simulink model "Xcvr_SSB_AM_2p5"  (Simulink 8.0)
settings: Solver=VariableStepDiscrete  SolverMode=SingleTasking  StartTime=0.0  StopTime=10  RelTol=1e-3
PreLoadFcn:
  | Fs=80e6;
  | 
  | phee=da_rom();
  | [phee_1,phee_2]=da_i2_rom();
  | 
  | Dcic=64;       % CIC decimation
  | Dfac=128;    % following DA filter decimation
  | N = 6;           %       (2^(N+1))=Dfac
  | Daudio=Dcic*Dfac;
  | Faudio=Fs/Daudio;
  | 
  | load info_filt_ssb_4
  | load Serial_Intfc_Stream_5
  | 
  | % AGC related
  | x=0.5:1/256:(1-1/256);
  | addr=(x-0.5)*256;
  | y=1./x;
values from neighbouring files (symbols this model uses):
  Serial_Interface = [0 0 0 0 0 0 0 0 0 0 0 0 ... (11390 elements, 2x5695)]    [Serial_Intfc_Stream_5.mat]
undefined symbols (not defined in the file or in its folder): get, sided, Two, xlipgetpartsetting
undefined symbols (not defined in the file): ssb_coef
libraries: xbsIndex_r4 x1305, dspsrcs4 x5, simulink x2, dspsigops x2, dspsnks4 x1
(part 11 of 11)

== system Xcvr_SSB_AM_2p5/Audio_and_Mode_Control/AGC_and_More/AGC Xilinx/Sequential Divide/Shift and lookup ==
  note: Delays to equalize for ROM latency.
  note: b16
  In1 : Inport
  1st 1 detect : Subsystem
  AddSub : xbsIndex_r4/AddSub  mode=Subtraction  use_carryin=off  use_carryout=off  en=off  latency=0  precision=User Defined  arith_type=Unsigned  n_bits=8  bin_pt=0  quantization=Truncate  overflow=Saturate  dbl_ovrd=off  use_behavioral_HDL=off  hw_selection=Fabric  pipelined=off  use_rpm=on  block_type=addsub
      settings: block_version=9.2.00
  AddSub1 : xbsIndex_r4/AddSub  mode=Addition  use_carryin=off  use_carryout=off  en=off  latency=0  precision=User Defined  arith_type=Unsigned  n_bits=8  bin_pt=0  quantization=Truncate  overflow=Saturate  dbl_ovrd=off  use_behavioral_HDL=off  hw_selection=Fabric  pipelined=off  use_rpm=on  block_type=addsub
      settings: block_version=9.2.00
  CMult : xbsIndex_r4/CMult  const=1/8  gui_display_data_type=Fixed-point  const_n_bits=3  const_bin_pt=3  float_type=Single  exp_bits=8  fraction_bits=24  en=off  latency=0  precision=User Defined  arith_type=Unsigned  n_bits=8  bin_pt=0  quantization=Truncate  overflow=Wrap  dbl_ovrd=off  use_behavioral_HDL=off  mem_type=Distributed RAM  pipeline=off  block_type=cmult
      settings: block_version=12.2
  CMult1 : xbsIndex_r4/CMult  const=16  gui_display_data_type=Fixed-point  const_n_bits=5  const_bin_pt=0  float_type=Single  exp_bits=8  fraction_bits=24  en=off  latency=0  precision=User Defined  arith_type=Unsigned  n_bits=8  bin_pt=0  quantization=Truncate  overflow=Wrap  dbl_ovrd=off  use_behavioral_HDL=off  mem_type=Distributed RAM  pipeline=off  block_type=cmult
      settings: block_version=12.2
  Capture Fraction and compute address : Subsystem
  Capture Shift : Subsystem
  Constant : xbsIndex_r4/Constant  const=0  gui_display_data_type=Fixed-point  arith_type=Unsigned  n_bits=5  bin_pt=0  preci_type=Single  exp_width=8  frac_width=24  explicit_period=off  period=1  equ=P=C  opselect=C  inp2=PCIN>>17  opr=+  inp1=P  carry=CIN  dbl_ovrd=off  block_type=constant
      settings: block_version=9.2.00
  Constant1 : xbsIndex_r4/Constant  const=16  gui_display_data_type=Fixed-point  arith_type=Unsigned  n_bits=5  bin_pt=0  preci_type=Single  exp_width=8  frac_width=24  explicit_period=off  period=1  equ=P=C  opselect=C  inp2=PCIN>>17  opr=+  inp1=P  carry=CIN  dbl_ovrd=off  block_type=constant
      settings: block_version=9.2.00
  Constant2 : xbsIndex_r4/Constant  const=15  gui_display_data_type=Fixed-point  arith_type=Unsigned  n_bits=4  bin_pt=0  preci_type=Single  exp_width=8  frac_width=24  explicit_period=off  period=1  equ=P=C  opselect=C  inp2=PCIN>>17  opr=+  inp1=P  carry=CIN  dbl_ovrd=off  block_type=constant
      settings: block_version=9.2.00
  Counter : xbsIndex_r4/Counter  cnt_type=Count Limited  cnt_to=31  operation=Up  start_count=0  cnt_by_val=1  arith_type=Unsigned  n_bits=5  bin_pt=0  load_pin=off  rst=off  en=off  explicit_period=on  period=1/(32*Faudio)  dbl_ovrd=off  use_behavioral_HDL=off  implementation=Fabric  use_rpm=off  block_type=counter
      settings: block_version=9.2.00
  Counter1 : xbsIndex_r4/Counter  cnt_type=Free Running  cnt_to=255  operation=Up  start_count=0  cnt_by_val=1  arith_type=Unsigned  n_bits=8  bin_pt=0  load_pin=off  rst=off  en=off  explicit_period=on  period=1/(32*Faudio)  dbl_ovrd=off  use_behavioral_HDL=off  implementation=Fabric  use_rpm=off  block_type=counter
      settings: block_version=9.2.00
  Delay1 : xbsIndex_r4/Delay  rst=off  infoeditControl=Selection of Reset will increase slice count due to use of real FFs and instead of SRLs  en=off  latency=1  dbl_ovrd=off  reg_retiming=off  block_type=delay
      settings: block_version=9.2.00
  Delay2 : xbsIndex_r4/Delay  rst=off  infoeditControl=Selection of Reset will increase slice count due to use of real FFs and instead of SRLs  en=off  latency=1  dbl_ovrd=off  reg_retiming=off  block_type=delay
      settings: block_version=9.2.00
  Mux : xbsIndex_r4/Mux  inputs=2  en=off  latency=1  precision=Full  arith_type=Unsigned  n_bits=16  bin_pt=14  quantization=Truncate  overflow=Wrap  dbl_ovrd=off  block_type=mux
      settings: block_version=9.2.00
  ROM : xbsIndex_r4/ROM  depth=128  initVector=y  distributed_mem=Block RAM  rst=off  init_reg=0  en=off  latency=1  gui_display_data_type=Fixed-point  arith_type=Unsigned  n_bits=10  bin_pt=9  preci_type=Single  exp_width=8  frac_width=24  dbl_ovrd=off  optimize=Area  use_rpm=on  block_type=sprom
      settings: block_version=9.2.00
  Relational : xbsIndex_r4/Relational  mode=a=b  en=off  latency=0  dbl_ovrd=off  block_type=relational
      settings: block_version=9.2.00
  Relational1 : xbsIndex_r4/Relational  mode=a=b  en=off  latency=0  dbl_ovrd=off  block_type=relational
      settings: block_version=9.2.00
  Relational3 : xbsIndex_r4/Relational  mode=a<b  en=off  latency=0  dbl_ovrd=off  block_type=relational
      settings: block_version=9.2.00
  Shift1 : xbsIndex_r4/Shift  shift_dir=Left  shift_bits=1  en=off  latency=0  precision=User Defined  arith_type=Unsigned  n_bits=16  bin_pt=16  quantization=Truncate  overflow=Wrap  dbl_ovrd=off  block_type=shift
      settings: block_version=9.2.00
  Slice : xbsIndex_r4/Slice  nbits=1  boolean_output=off  mode=Upper Bit Location + Width  bit1=0  base1=MSB of Input  bit0=0  base0=LSB of Input  dbl_ovrd=off  block_type=slice
      settings: infoedit="Extracts a given range of bits from each input sample and presents it at the output.  The output type is ordinarily unsigned with binary point at zero, but can be Boolean when the slice is one bit wide.<P><P>Hardware notes: In hardware this block costs nothing."  block_version=9.2.00
  Ready : Outport
  1/X : Outport  Port=2
  Shift : Outport  Port=3
  Smeter : Outport  Port=4
  wires:
  Delay1/1 -> Ready/1
  ROM/1 -> 1/X/1
  Capture Shift/1(Dout) -> Delay2/1
  Capture Fraction and compute address/1(Dout) -> CMult/1, ROM/1
  1st 1 detect/1(Out1) -> Capture Shift/1(En), Capture Fraction and compute address/2(En)
  Slice/1 -> 1st 1 detect/1(MSbit)
  Relational1/1 -> Delay1/1
  Constant1/1 -> Relational1/2
  Constant/1 -> Relational/2
  Counter/1 -> Capture Shift/2(Din), Relational1/1, Relational/1
  In1/1 -> Mux/3
  Shift1/1 -> Mux/2
  Relational/1 -> 1st 1 detect/2(Rst), Mux/1
  Mux/1 -> Shift1/1, Slice/1, Capture Fraction and compute address/1(Din)
  CMult/1 -> AddSub/2
  AddSub/1 -> Relational3/1
  AddSub1/1 -> AddSub/1
  CMult1/1 -> AddSub1/2
  Constant2/1 -> AddSub1/1
  Delay2/1 -> CMult1/1, Shift/1
  Counter1/1 -> Relational3/2
  Relational3/1 -> Smeter/1  "Uncorrected"

== system Xcvr_SSB_AM_2p5/Audio_and_Mode_Control/AGC_and_More/AGC Xilinx/Sequential Divide/Variable Shifter ==
  EN : Inport
  Din : Inport  Port=2
  Shift in : Inport  Port=3
  Mux : xbsIndex_r4/Mux  inputs=16  en=on  latency=1  precision=Full  arith_type=Unsigned  n_bits=16  bin_pt=14  quantization=Truncate  overflow=Wrap  dbl_ovrd=off  block_type=mux
      settings: block_version=9.2.00
  Shift{1..15} (15 alike) : xbsIndex_r4/Shift  shift_dir=Left  shift_bits=1  en=off  latency=0  precision=Full  arith_type="Signed  (2's comp)"  n_bits=16  bin_pt=14  quantization=Truncate  overflow=Wrap  dbl_ovrd=off  block_type=shift
      settings: block_version=9.2.00
  Out1 : Outport
  wires:
  Shift15/1 -> Mux/17
  Shift14/1 -> Shift15/1, Mux/16
  Shift13/1 -> Shift14/1, Mux/15
  Shift12/1 -> Shift13/1, Mux/14
  Shift11/1 -> Shift12/1, Mux/13
  Shift10/1 -> Shift11/1, Mux/12
  Shift9/1 -> Shift10/1, Mux/11
  Shift8/1 -> Shift9/1, Mux/10
  Shift7/1 -> Shift8/1, Mux/9
  Shift6/1 -> Shift7/1, Mux/8
  Shift5/1 -> Shift6/1, Mux/7
  Shift4/1 -> Shift5/1, Mux/6
  Shift3/1 -> Shift4/1, Mux/5
  Shift2/1 -> Shift3/1, Mux/4
  Shift1/1 -> Shift2/1, Mux/3
  EN/1 -> Mux/18
  Mux/1 -> Out1/1
  Din/1 -> Shift1/1, Mux/2
  Shift in/1 -> Mux/1

== system Xcvr_SSB_AM_2p5/Audio_and_Mode_Control/AGC_and_More/RX_Audio_Filter/n-tap MAC FIR Filter/MAC Engine ==
  note: The precision required for the multiplier and the accumulator is a
      | function of the filter taps (coefficients) and the number of taps. Since
      | these are fixed at design time, it is possible to tailor the hardware resources
      | to the filter specification.  The multiplier need only have enough  bits to
      | compute the product of the largest magnitude coefficient and the largest
      | magnitude data input value.   That is,
      |
      |         mult_nbits = ceil(log2(max(abs(coef*2^coef_binpt))))+input_nbits + 1;
      |         mult_binpt = input_binpt+coef_binpt;
      |
      | Similarly, the accumulator need only have sufficient precision to accumulate
      | maximal input against the filter taps.
      |
      |         acc_nbits = ceil(log2(sum(abs(coef*2^coef_binpt)))) + input_nbits + 1;
      |         acc_binpt = mult_binpt;
      |
      | These variables are passed to the blocks as mask parameters.
  note: Upon reset, the accumulator reinitializes to its current input value
      | rather than zero, which allows the MAC engine to stream data without
      | stalling for one sample period.
  note: This subsystem implements a multiply-accumulate engine.
  note: The Multiplier block is implemented using Virtex-II  dedicated multipliers.
      | Enabling the 'Pipeline to Greatest Extent Possible' mask configuration
      | parameter ensures the internal pipeline stages of the dedicated
      | multipliers are used.
  a : Inport
  b : Inport  Port=2
  rst : Inport  Port=3
  Accumulator : xbsIndex_r4/Accumulator  operation=Add  n_bits=ceil(log2(max(1,sum(abs(coef*2^coef_bin_pt)))))+smpl_n_bits + 1  overflow=Wrap  scale=1  rst=on  infoeditControl=reset for floating point data type must be asserted for a minimum of 2 cycles  hasbypass=on  en=off  latency=0  dbl_ovrd=off  msb_inp=100  msb=100  lsb=-100  use_behavioral_HDL=on  implementation=Fabric  block_type=accum
      settings: infoedit="Adder or subtractor-based accumulator.   Output type and binary point position match the input.<P><P>Hardware notes: When \"Reinitialize with Input 'b' on Reset\" is selected, the accumulator is forced to run at the system rate even if the input 'b' is running at a slower rate."  xl_area=[0, 0, 0, 0, 0, 0, 0]  block_version=VER_STRING_GOES_HERE
  Mult : xbsIndex_r4/Mult  precision=User Defined  arith_type="Signed  (2's comp)"  n_bits=max(ceil(log2(max(1,max(abs(coef*2^coef_bin_pt)))))+smpl_n_bits + 1,smpl_bin_pt+coef_bin_pt)  bin_pt=smpl_bin_pt+coef_bin_pt  quantization=Truncate  overflow=Wrap  en=off  latency=2  dbl_ovrd=off  use_behavioral_HDL=off  opt=Speed  use_embedded=on  optimum_pipeline=off  pipeline=on  use_rpm=on  placement_style=Rectangular shape  block_type=mult
      settings: infoedit=Multiplies two values.<P><P>Hardware notes: To use the internal pipeline stage of the dedicated multiplier you must select 'Pipeline to Greatest Extent Possible'.  xl_area=[0, 0, 0, 0, 0, 0, 0]  block_version=VER_STRING_GOES_HERE
  q : Outport
  wires:
  Mult/1 -> Accumulator/1
  a/1 -> Mult/1
  Accumulator/1 -> q/1
  b/1 -> Mult/2
  rst/1 -> Accumulator/2

== system Xcvr_SSB_AM_2p5/Audio_and_Mode_Control/Audio_Processor/TX Equalizer/n-tap MAC FIR Filter/MAC Engine ==
  note: The precision required for the multiplier and the accumulator is a
      | function of the filter taps (coefficients) and the number of taps. Since
      | these are fixed at design time, it is possible to tailor the hardware resources
      | to the filter specification.  The multiplier need only have enough  bits to
      | compute the product of the largest magnitude coefficient and the largest
      | magnitude data input value.   That is,
      |
      |         mult_nbits = ceil(log2(max(abs(coef*2^coef_binpt))))+input_nbits + 1;
      |         mult_binpt = input_binpt+coef_binpt;
      |
      | Similarly, the accumulator need only have sufficient precision to accumulate
      | maximal input against the filter taps.
      |
      |         acc_nbits = ceil(log2(sum(abs(coef*2^coef_binpt)))) + input_nbits + 1;
      |         acc_binpt = mult_binpt;
      |
      | These variables are passed to the blocks as mask parameters.
  note: Upon reset, the accumulator reinitializes to its current input value
      | rather than zero, which allows the MAC engine to stream data without
      | stalling for one sample period.
  note: This subsystem implements a multiply-accumulate engine.
  note: The Multiplier block is implemented using Virtex-II  dedicated multipliers.
      | Enabling the 'Pipeline to Greatest Extent Possible' mask configuration
      | parameter ensures the internal pipeline stages of the dedicated
      | multipliers are used.
  a : Inport
  b : Inport  Port=2
  rst : Inport  Port=3
  Accumulator : xbsIndex_r4/Accumulator  operation=Add  n_bits=ceil(log2(max(1,sum(abs(coef*2^coef_bin_pt)))))+smpl_n_bits + 1  overflow=Wrap  scale=1  rst=on  infoeditControl=reset for floating point data type must be asserted for a minimum of 2 cycles  hasbypass=on  en=off  latency=0  dbl_ovrd=off  msb_inp=100  msb=100  lsb=-100  use_behavioral_HDL=on  implementation=Fabric  block_type=accum
      settings: infoedit="Adder or subtractor-based accumulator.   Output type and binary point position match the input.<P><P>Hardware notes: When \"Reinitialize with Input 'b' on Reset\" is selected, the accumulator is forced to run at the system rate even if the input 'b' is running at a slower rate."  xl_area=[0, 0, 0, 0, 0, 0, 0]  block_version=VER_STRING_GOES_HERE
  Mult : xbsIndex_r4/Mult  precision=User Defined  arith_type="Signed  (2's comp)"  n_bits=max(ceil(log2(max(1,max(abs(coef*2^coef_bin_pt)))))+smpl_n_bits + 1,smpl_bin_pt+coef_bin_pt)  bin_pt=smpl_bin_pt+coef_bin_pt  quantization=Truncate  overflow=Wrap  en=off  latency=2  dbl_ovrd=off  use_behavioral_HDL=off  opt=Speed  use_embedded=on  optimum_pipeline=off  pipeline=on  use_rpm=on  placement_style=Rectangular shape  block_type=mult
      settings: infoedit=Multiplies two values.<P><P>Hardware notes: To use the internal pipeline stage of the dedicated multiplier you must select 'Pipeline to Greatest Extent Possible'.  xl_area=[0, 0, 0, 0, 0, 0, 0]  block_version=VER_STRING_GOES_HERE
  q : Outport
  wires:
  Mult/1 -> Accumulator/1
  a/1 -> Mult/1
  Accumulator/1 -> q/1
  b/1 -> Mult/2
  rst/1 -> Accumulator/2

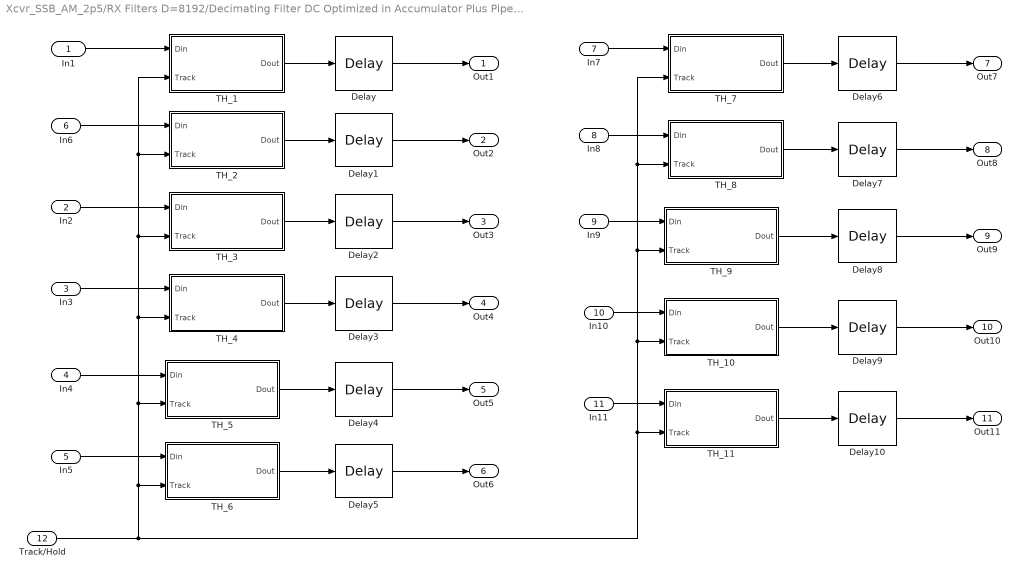
== system Xcvr_SSB_AM_2p5/RX Filters D=8192/Decimating Filter DC Optimized in Accumulator Plus Pipelined Stage Control. Improved dynamic  range. /D=2 Bit Serial Filter Core with Piplined RAM Based SR/RAM Based SR/Track/Hang  Plus 1 Pipe Stage ==
  In1 : Inport
  In2 : Inport  Port=2
  In3 : Inport  Port=3
  In4 : Inport  Port=4
  In5 : Inport  Port=5
  In6 : Inport  Port=6
  In7 : Inport  Port=7
  In8 : Inport  Port=8
  In9 : Inport  Port=9
  In10 : Inport  Port=10
  In11 : Inport  Port=11
  Track/Hold : Inport  Port=12
  Delay{,1..10} (11 alike) : xbsIndex_r4/Delay  rst=off  infoeditControl=Selection of Reset will increase slice count due to use of real FFs and instead of SRLs  en=off  latency=1  dbl_ovrd=off  reg_retiming=off  block_type=delay
      settings: block_version=12.2
  TH_1 : Subsystem
  TH_10 : Subsystem
  TH_11 : Subsystem
  TH_2 : Subsystem
  TH_3 : Subsystem
  TH_4 : Subsystem
  TH_5 : Subsystem
  TH_6 : Subsystem
  TH_7 : Subsystem
  TH_8 : Subsystem
  TH_9 : Subsystem
  Out1 : Outport
  Out2 : Outport  Port=2
  Out3 : Outport  Port=3
  Out4 : Outport  Port=4
  Out5 : Outport  Port=5
  Out6 : Outport  Port=6
  Out7 : Outport  Port=7
  Out8 : Outport  Port=8
  Out9 : Outport  Port=9
  Out10 : Outport  Port=10
  Out11 : Outport  Port=11
  wires:
  TH_5/1(Dout) -> Delay4/1
  TH_8/1(Dout) -> Delay7/1
  TH_9/1(Dout) -> Delay8/1
  TH_10/1(Dout) -> Delay9/1
  TH_2/1(Dout) -> Delay1/1
  In9/1 -> TH_9/1(Din)
  In10/1 -> TH_10/1(Din)
  In5/1 -> TH_6/1(Din)
  TH_4/1(Dout) -> Delay3/1
  In6/1 -> TH_2/1(Din)
  In7/1 -> TH_7/1(Din)
  In4/1 -> TH_5/1(Din)
  In8/1 -> TH_8/1(Din)
  In1/1 -> TH_1/1(Din)
  In3/1 -> TH_4/1(Din)
  In2/1 -> TH_3/1(Din)
  TH_1/1(Dout) -> Delay/1
  In11/1 -> TH_11/1(Din)
  TH_11/1(Dout) -> Delay10/1
  TH_7/1(Dout) -> Delay6/1
  TH_6/1(Dout) -> Delay5/1
  TH_3/1(Dout) -> Delay2/1
  Delay/1 -> Out1/1
  Delay1/1 -> Out2/1
  Delay2/1 -> Out3/1
  Delay3/1 -> Out4/1
  Delay4/1 -> Out5/1
  Delay5/1 -> Out6/1
  Delay6/1 -> Out7/1
  Delay7/1 -> Out8/1
  Delay8/1 -> Out9/1
  Delay9/1 -> Out10/1
  Delay10/1 -> Out11/1
  Track/Hold/1 -> TH_6/2(Track), TH_5/2(Track), TH_4/2(Track), TH_3/2(Track), TH_1/2(Track), TH_2/2(Track), TH_7/2(Track), TH_8/2(Track), TH_9/2(Track), TH_10/2(Track), TH_11/2(Track)

== system Xcvr_SSB_AM_2p5/RX Filters D=8192/Decimating Filter DC Optimized in Accumulator Plus Pipelined Stage Control. Improved dynamic  range. /D=2 Bit Serial Filter Core with Piplined RAM Based SR/SAD_1/Full Adder ==
  note: Full Adder Logic
  A : Inport
  B : Inport  Port=2
  Cin : Inport  Port=3
  Logical : xbsIndex_r4/Logical  logical_function=AND  inputs=2  en=off  latency=0  precision=Full  arith_type=Unsigned  n_bits=16  bin_pt=0  align_bp=on  dbl_ovrd=off  block_type=logical
      settings: block_version=9.2.00
  Logical1 : xbsIndex_r4/Logical  logical_function=AND  inputs=2  en=off  latency=0  precision=Full  arith_type=Unsigned  n_bits=16  bin_pt=0  align_bp=on  dbl_ovrd=off  block_type=logical
      settings: block_version=9.2.00
  Logical2 : xbsIndex_r4/Logical  logical_function=OR  inputs=2  en=off  latency=0  precision=Full  arith_type=Unsigned  n_bits=16  bin_pt=0  align_bp=on  dbl_ovrd=off  block_type=logical
      settings: block_version=9.2.00
  Logical3 : xbsIndex_r4/Logical  logical_function=XOR  inputs=2  en=off  latency=0  precision=Full  arith_type=Unsigned  n_bits=16  bin_pt=0  align_bp=on  dbl_ovrd=off  block_type=logical
      settings: block_version=9.2.00
  Logical4 : xbsIndex_r4/Logical  logical_function=XOR  inputs=2  en=off  latency=0  precision=Full  arith_type=Unsigned  n_bits=16  bin_pt=0  align_bp=on  dbl_ovrd=off  block_type=logical
      settings: block_version=9.2.00
  Sum : Outport
  Cout : Outport  Port=2
  wires:
  Logical3/1 -> Logical1/2, Logical4/1
  Cin/1 -> Logical1/1, Logical4/2
  B/1 -> Logical/2, Logical3/2
  A/1 -> Logical/1, Logical3/1
  Logical/1 -> Logical2/2
  Logical1/1 -> Logical2/1
  Logical4/1 -> Sum/1  "Sout"
  Logical2/1 -> Cout/1  "Cout"

== system Xcvr_SSB_AM_2p5/RX Filters D=8192/Decimating Filter DC Optimized in Accumulator Plus Pipelined Stage Control. Improved dynamic  range. /D=2 Bit Serial Filter Core with Piplined RAM Based SR/SAD_2/Full Adder ==
  note: Full Adder Logic
  A : Inport
  B : Inport  Port=2
  Cin : Inport  Port=3
  Logical : xbsIndex_r4/Logical  logical_function=AND  inputs=2  en=off  latency=0  precision=Full  arith_type=Unsigned  n_bits=16  bin_pt=0  align_bp=on  dbl_ovrd=off  block_type=logical
      settings: block_version=9.2.00
  Logical1 : xbsIndex_r4/Logical  logical_function=AND  inputs=2  en=off  latency=0  precision=Full  arith_type=Unsigned  n_bits=16  bin_pt=0  align_bp=on  dbl_ovrd=off  block_type=logical
      settings: block_version=9.2.00
  Logical2 : xbsIndex_r4/Logical  logical_function=OR  inputs=2  en=off  latency=0  precision=Full  arith_type=Unsigned  n_bits=16  bin_pt=0  align_bp=on  dbl_ovrd=off  block_type=logical
      settings: block_version=9.2.00
  Logical3 : xbsIndex_r4/Logical  logical_function=XOR  inputs=2  en=off  latency=0  precision=Full  arith_type=Unsigned  n_bits=16  bin_pt=0  align_bp=on  dbl_ovrd=off  block_type=logical
      settings: block_version=9.2.00
  Logical4 : xbsIndex_r4/Logical  logical_function=XOR  inputs=2  en=off  latency=0  precision=Full  arith_type=Unsigned  n_bits=16  bin_pt=0  align_bp=on  dbl_ovrd=off  block_type=logical
      settings: block_version=9.2.00
  Sum : Outport
  Cout : Outport  Port=2
  wires:
  Logical2/1 -> Cout/1  "Cout"
  Logical4/1 -> Sum/1  "Sout"
  Logical1/1 -> Logical2/1
  Logical/1 -> Logical2/2
  A/1 -> Logical3/1, Logical/1
  B/1 -> Logical3/2, Logical/2
  Cin/1 -> Logical4/2, Logical1/1
  Logical3/1 -> Logical4/1, Logical1/2

== system Xcvr_SSB_AM_2p5/RX Filters D=8192/Decimating Filter DC Optimized in Accumulator Plus Pipelined Stage Control. Improved dynamic  range. /D=2 Bit Serial Filter Core with Piplined RAM Based SR/SAD_3/Full Adder ==
  note: Full Adder Logic
  A : Inport
  B : Inport  Port=2
  Cin : Inport  Port=3
  Logical : xbsIndex_r4/Logical  logical_function=AND  inputs=2  en=off  latency=0  precision=Full  arith_type=Unsigned  n_bits=16  bin_pt=0  align_bp=on  dbl_ovrd=off  block_type=logical
      settings: block_version=9.2.00
  Logical1 : xbsIndex_r4/Logical  logical_function=AND  inputs=2  en=off  latency=0  precision=Full  arith_type=Unsigned  n_bits=16  bin_pt=0  align_bp=on  dbl_ovrd=off  block_type=logical
      settings: block_version=9.2.00
  Logical2 : xbsIndex_r4/Logical  logical_function=OR  inputs=2  en=off  latency=0  precision=Full  arith_type=Unsigned  n_bits=16  bin_pt=0  align_bp=on  dbl_ovrd=off  block_type=logical
      settings: block_version=9.2.00
  Logical3 : xbsIndex_r4/Logical  logical_function=XOR  inputs=2  en=off  latency=0  precision=Full  arith_type=Unsigned  n_bits=16  bin_pt=0  align_bp=on  dbl_ovrd=off  block_type=logical
      settings: block_version=9.2.00
  Logical4 : xbsIndex_r4/Logical  logical_function=XOR  inputs=2  en=off  latency=0  precision=Full  arith_type=Unsigned  n_bits=16  bin_pt=0  align_bp=on  dbl_ovrd=off  block_type=logical
      settings: block_version=9.2.00
  Sum : Outport
  Cout : Outport  Port=2
  wires:
  Logical3/1 -> Logical1/2, Logical4/1
  Cin/1 -> Logical1/1, Logical4/2
  B/1 -> Logical/2, Logical3/2
  A/1 -> Logical/1, Logical3/1
  Logical/1 -> Logical2/2
  Logical1/1 -> Logical2/1
  Logical4/1 -> Sum/1  "Sout"
  Logical2/1 -> Cout/1  "Cout"

== system Xcvr_SSB_AM_2p5/RX Filters D=8192/Decimating Filter DC Optimized in Accumulator Plus Pipelined Stage Control. Improved dynamic  range. /D=2 Bit Serial Filter Core with Piplined RAM Based SR/SAD_4/Full Adder ==
  note: Full Adder Logic
  A : Inport
  B : Inport  Port=2
  Cin : Inport  Port=3
  Logical : xbsIndex_r4/Logical  logical_function=AND  inputs=2  en=off  latency=0  precision=Full  arith_type=Unsigned  n_bits=16  bin_pt=0  align_bp=on  dbl_ovrd=off  block_type=logical
      settings: block_version=9.2.00
  Logical1 : xbsIndex_r4/Logical  logical_function=AND  inputs=2  en=off  latency=0  precision=Full  arith_type=Unsigned  n_bits=16  bin_pt=0  align_bp=on  dbl_ovrd=off  block_type=logical
      settings: block_version=9.2.00
  Logical2 : xbsIndex_r4/Logical  logical_function=OR  inputs=2  en=off  latency=0  precision=Full  arith_type=Unsigned  n_bits=16  bin_pt=0  align_bp=on  dbl_ovrd=off  block_type=logical
      settings: block_version=9.2.00
  Logical3 : xbsIndex_r4/Logical  logical_function=XOR  inputs=2  en=off  latency=0  precision=Full  arith_type=Unsigned  n_bits=16  bin_pt=0  align_bp=on  dbl_ovrd=off  block_type=logical
      settings: block_version=9.2.00
  Logical4 : xbsIndex_r4/Logical  logical_function=XOR  inputs=2  en=off  latency=0  precision=Full  arith_type=Unsigned  n_bits=16  bin_pt=0  align_bp=on  dbl_ovrd=off  block_type=logical
      settings: block_version=9.2.00
  Sum : Outport
  Cout : Outport  Port=2
  wires:
  Logical2/1 -> Cout/1  "Cout"
  Logical4/1 -> Sum/1  "Sout"
  Logical1/1 -> Logical2/1
  Logical/1 -> Logical2/2
  A/1 -> Logical3/1, Logical/1
  B/1 -> Logical3/2, Logical/2
  Cin/1 -> Logical4/2, Logical1/1
  Logical3/1 -> Logical4/1, Logical1/2

== system Xcvr_SSB_AM_2p5/RX Filters D=8192/Decimating Filter DC Optimized in Accumulator Plus Pipelined Stage Control. Improved dynamic  range. /D=2 Bit Serial Filter Core with Piplined RAM Based SR/Timing/Control1/S-R FF1 ==
  Set : Inport
  Reset : Inport  Port=2
  Logical : xbsIndex_r4/Logical  logical_function=OR  inputs=2  en=off  latency=0  precision=Full  arith_type=Unsigned  n_bits=16  bin_pt=0  align_bp=on  dbl_ovrd=off  block_type=logical
      settings: block_version=VER_STRING_GOES_HERE
  Register : xbsIndex_r4/Register  init=0  rst=on  en=off  dbl_ovrd=off  block_type=register
      settings: block_version=VER_STRING_GOES_HERE
  Q : Outport
  wires:
  Reset/1 -> Register/2
  Set/1 -> Logical/2
  Register/1 -> Logical/1
  Logical/1 -> Q/1, Register/1

== system Xcvr_SSB_AM_2p5/RX Filters D=8192/Decimating Filter DC Optimized in Accumulator Plus Pipelined Stage Control. Improved dynamic  range. /Stage Control with Pipe/Stage_Control/Priority_Encoder ==
  In1 : Inport
  In2 : Inport  Port=2
  In3 : Inport  Port=3
  In4 : Inport  Port=4
  In5 : Inport  Port=5
  In6 : Inport  Port=6
  In7 : Inport  Port=7
  Inverter{,1..6} (7 alike) : xbsIndex_r4/Inverter  en=off  latency=0  dbl_ovrd=off  block_type=inv
      settings: block_version=9.2.00
  Logical : xbsIndex_r4/Logical  logical_function=AND  inputs=4  en=off  latency=0  precision=Full  arith_type=Unsigned  n_bits=16  bin_pt=0  align_bp=on  dbl_ovrd=off  block_type=logical
      settings: block_version=9.2.00
  Logical1 : xbsIndex_r4/Logical  logical_function=NOR  inputs=4  en=off  latency=0  precision=Full  arith_type=Unsigned  n_bits=16  bin_pt=0  align_bp=on  dbl_ovrd=off  block_type=logical
      settings: block_version=9.2.00
  Logical2 : xbsIndex_r4/Logical  logical_function=AND  inputs=3  en=off  latency=0  precision=Full  arith_type=Unsigned  n_bits=16  bin_pt=0  align_bp=on  dbl_ovrd=off  block_type=logical
      settings: block_version=9.2.00
  Logical3 : xbsIndex_r4/Logical  logical_function=AND  inputs=2  en=off  latency=0  precision=Full  arith_type=Unsigned  n_bits=16  bin_pt=0  align_bp=on  dbl_ovrd=off  block_type=logical
      settings: block_version=9.2.00
  Logical4 : xbsIndex_r4/Logical  logical_function=AND  inputs=3  en=off  latency=0  precision=Full  arith_type=Unsigned  n_bits=16  bin_pt=0  align_bp=on  dbl_ovrd=off  block_type=logical
      settings: block_version=9.2.00
  Logical5 : xbsIndex_r4/Logical  logical_function=AND  inputs=3  en=off  latency=0  precision=Full  arith_type=Unsigned  n_bits=16  bin_pt=0  align_bp=on  dbl_ovrd=off  block_type=logical
      settings: block_version=9.2.00
  Logical6 : xbsIndex_r4/Logical  logical_function=NOR  inputs=4  en=off  latency=0  precision=Full  arith_type=Unsigned  n_bits=16  bin_pt=0  align_bp=on  dbl_ovrd=off  block_type=logical
      settings: block_version=9.2.00
  Logical7 : xbsIndex_r4/Logical  logical_function=NOR  inputs=4  en=off  latency=0  precision=Full  arith_type=Unsigned  n_bits=16  bin_pt=0  align_bp=on  dbl_ovrd=off  block_type=logical
      settings: block_version=9.2.00
  Out1 : Outport
  Out2 : Outport  Port=2
  Out3 : Outport  Port=3
  wires:
  Inverter/1 -> Logical/1
  Logical/1 -> Logical1/1
  Logical2/1 -> Logical1/2
  Logical3/1 -> Logical1/3
  Logical4/1 -> Logical6/1
  Logical5/1 -> Logical6/2
  In2/1 -> Inverter1/1, Logical/2
  In4/1 -> Inverter3/1, Logical/3, Logical2/2, Logical4/2, Logical5/2
  In5/1 -> Inverter4/1, Logical4/3, Logical5/3
  In6/1 -> Inverter5/1, Logical/4, Logical2/3, Logical3/2
  Inverter2/1 -> Logical2/1, Logical5/1
  Inverter1/1 -> Logical4/1
  Inverter5/1 -> Logical6/3, Logical7/3
  Inverter6/1 -> Logical7/4, Logical6/4, Logical1/4
  Inverter4/1 -> Logical7/2, Logical3/1
  Inverter3/1 -> Logical7/1
  In1/1 -> Inverter/1
  In3/1 -> Inverter2/1
  Logical1/1 -> Out1/1
  In7/1 -> Inverter6/1
  Logical6/1 -> Out2/1
  Logical7/1 -> Out3/1

== system Xcvr_SSB_AM_2p5/Audio_and_Mode_Control/AGC_and_More/AGC Xilinx/Sequential Divide/Shift and lookup/1st 1 detect ==
  note: Capture 1st MSbit change from 0 to 1 and produce a pulse.
  MSbit : Inport
  Rst : Inport  Port=2
  Constant : xbsIndex_r4/Constant  const=0  gui_display_data_type=Fixed-point  arith_type=Unsigned  n_bits=1  bin_pt=0  preci_type=Single  exp_width=8  frac_width=24  explicit_period=off  period=1  equ=P=C  opselect=C  inp2=PCIN>>17  opr=+  inp1=P  carry=CIN  dbl_ovrd=off  block_type=constant
      settings: block_version=9.2.00
  Convert : xbsIndex_r4/Convert  gui_display_data_type=Fixed-point  arith_type=Boolean  n_bits=16  bin_pt=14  float_type=Single  exp_bits=8  fraction_bits=24  quantization=Truncate  overflow=Wrap  en=off  latency=0  dbl_ovrd=off  pipeline=off  block_type=convert
      settings: block_version=9.2.00
  Delay : xbsIndex_r4/Delay  rst=off  infoeditControl=Selection of Reset will increase slice count due to use of real FFs and instead of SRLs  en=off  latency=1  dbl_ovrd=off  reg_retiming=off  block_type=delay
      settings: block_version=9.2.00
  Inverter : xbsIndex_r4/Inverter  en=off  latency=0  dbl_ovrd=off  block_type=inv
      settings: block_version=9.2.00
  Logical : xbsIndex_r4/Logical  logical_function=AND  inputs=2  en=off  latency=0  precision=Full  arith_type=Unsigned  n_bits=16  bin_pt=0  align_bp=on  dbl_ovrd=off  block_type=logical
      settings: block_version=9.2.00
  Logical1 : xbsIndex_r4/Logical  logical_function=OR  inputs=2  en=off  latency=0  precision=Full  arith_type=Unsigned  n_bits=16  bin_pt=0  align_bp=on  dbl_ovrd=off  block_type=logical
      settings: block_version=9.2.00
  Mux : xbsIndex_r4/Mux  inputs=2  en=off  latency=0  precision=User Defined  arith_type=Unsigned  n_bits=1  bin_pt=0  quantization=Truncate  overflow=Wrap  dbl_ovrd=off  block_type=mux
      settings: block_version=9.2.00
  Register : xbsIndex_r4/Register  init=0  rst=on  en=off  dbl_ovrd=off  block_type=register
      settings: block_version=9.2.00
  Out1 : Outport
  wires:
  Convert/1 -> Logical/1, Delay/1
  Rst/1 -> Register/2
  Register/1 -> Mux/1, Logical1/1
  Logical1/1 -> Register/1
  Logical/1 -> Logical1/2, Out1/1
  Inverter/1 -> Logical/2
  Delay/1 -> Inverter/1
  Mux/1 -> Convert/1
  MSbit/1 -> Mux/2
  Constant/1 -> Mux/3

== system Xcvr_SSB_AM_2p5/Audio_and_Mode_Control/AGC_and_More/AGC Xilinx/Sequential Divide/Shift and lookup/Capture Fraction and compute address ==
  note: 0...127
  Din : Inport
  En : Inport  Port=2
  AddSub : xbsIndex_r4/AddSub  mode=Subtraction  use_carryin=off  use_carryout=off  en=off  latency=0  precision=User Defined  arith_type=Unsigned  n_bits=8  bin_pt=8  quantization=Truncate  overflow=Wrap  dbl_ovrd=off  use_behavioral_HDL=off  hw_selection=Fabric  pipelined=off  use_rpm=on  block_type=addsub
      settings: block_version=9.2.00
  Constant : xbsIndex_r4/Constant  const=.5  gui_display_data_type=Fixed-point  arith_type=Unsigned  n_bits=2  bin_pt=1  preci_type=Single  exp_width=8  frac_width=24  explicit_period=off  period=1  equ=P=C  opselect=C  inp2=PCIN>>17  opr=+  inp1=P  carry=CIN  dbl_ovrd=off  block_type=constant
      settings: block_version=9.2.00
  Convert : xbsIndex_r4/Convert  gui_display_data_type=Fixed-point  arith_type=Unsigned  n_bits=7  bin_pt=7  float_type=Single  exp_bits=8  fraction_bits=24  quantization=Truncate  overflow=Wrap  en=off  latency=0  dbl_ovrd=off  pipeline=off  block_type=convert
      settings: block_version=12.1
  Register : xbsIndex_r4/Register  init=0  rst=off  en=on  dbl_ovrd=off  block_type=register
      settings: block_version=12.1
  Reinterpret : xbsIndex_r4/Reinterpret  force_arith_type=on  arith_type=Unsigned  force_bin_pt=on  bin_pt=0  block_type=reinterpret
      settings: infoedit="Changes signal type without altering the binary representation.   You can changed the signal between signed and unsigned, and relocate the binary point.<P><P>Hardware notes: In hardware this block costs nothing.<P><P>Example:  Suppose the input is 6 bits wide, signed, with 2 fractional bits, and the output is forced to unsigned with 0 fractional bits.  Then an input of -2.0 (1110.00 in binary 2's complement) becomes an output of 56 (111000 in binary)."  block_version=9.2.00
  Shift : xbsIndex_r4/Shift  shift_dir=Left  shift_bits=1  en=off  latency=0  precision=Full  arith_type="Signed  (2's comp)"  n_bits=16  bin_pt=14  quantization=Truncate  overflow=Wrap  dbl_ovrd=off  block_type=shift
      settings: block_version=9.2.00
  Dout : Outport
  wires:
  Shift/1 -> Convert/1
  Din/1 -> Register/1
  Reinterpret/1 -> Dout/1
  Constant/1 -> AddSub/2
  AddSub/1 -> Shift/1
  En/1 -> Register/2
  Register/1 -> AddSub/1
  Convert/1 -> Reinterpret/1

== system Xcvr_SSB_AM_2p5/Audio_and_Mode_Control/AGC_and_More/AGC Xilinx/Sequential Divide/Shift and lookup/Capture Shift ==
  En : Inport
  Din : Inport  Port=2
  AddSub : xbsIndex_r4/AddSub  mode=Subtraction  use_carryin=off  use_carryout=off  en=off  latency=0  precision=User Defined  arith_type=Unsigned  n_bits=5  bin_pt=0  quantization=Truncate  overflow=Wrap  dbl_ovrd=off  use_behavioral_HDL=off  hw_selection=Fabric  pipelined=off  use_rpm=on  block_type=addsub
      settings: block_version=9.2.00
  Constant : xbsIndex_r4/Constant  const=1  gui_display_data_type=Fixed-point  arith_type=Unsigned  n_bits=5  bin_pt=0  preci_type=Single  exp_width=8  frac_width=24  explicit_period=off  period=1  equ=P=C  opselect=C  inp2=PCIN>>17  opr=+  inp1=P  carry=CIN  dbl_ovrd=off  block_type=constant
      settings: block_version=9.2.00
  Delay : xbsIndex_r4/Delay  rst=off  infoeditControl=Selection of Reset will increase slice count due to use of real FFs and instead of SRLs  en=off  latency=1  dbl_ovrd=off  reg_retiming=off  block_type=delay
      settings: block_version=9.2.00
  Mux1 : xbsIndex_r4/Mux  inputs=2  en=off  latency=0  precision=User Defined  arith_type=Unsigned  n_bits=5  bin_pt=0  quantization=Truncate  overflow=Wrap  dbl_ovrd=off  block_type=mux
      settings: block_version=9.2.00
  Dout : Outport
  wires:
  Din/1 -> Mux1/3
  Delay/1 -> Mux1/2
  Constant/1 -> AddSub/2
  AddSub/1 -> Dout/1
  Mux1/1 -> AddSub/1, Delay/1
  En/1 -> Mux1/1

== system Xcvr_SSB_AM_2p5/RX Filters D=8192/Decimating Filter DC Optimized in Accumulator Plus Pipelined Stage Control. Improved dynamic  range. /D=2 Bit Serial Filter Core with Piplined RAM Based SR/RAM Based SR/Track/Hang  Plus 1 Pipe Stage/TH_1 ==
  Din : Inport
  Track : Inport  Port=2
  Delay : xbsIndex_r4/Delay  rst=off  infoeditControl=Selection of Reset will increase slice count due to use of real FFs and instead of SRLs  en=off  latency=1  dbl_ovrd=off  reg_retiming=off  block_type=delay
      settings: block_version=12.2
  Mux : xbsIndex_r4/Mux  inputs=2  en=off  latency=0  precision=Full  arith_type=Unsigned  n_bits=16  bin_pt=14  quantization=Truncate  overflow=Wrap  dbl_ovrd=off  block_type=mux
      settings: block_version=12.2
  Dout : Outport
  wires:
  Mux/1 -> Dout/1
  Din/1 -> Delay/1, Mux/3
  Delay/1 -> Mux/2
  Track/1 -> Mux/1

== system Xcvr_SSB_AM_2p5/RX Filters D=8192/Decimating Filter DC Optimized in Accumulator Plus Pipelined Stage Control. Improved dynamic  range. /D=2 Bit Serial Filter Core with Piplined RAM Based SR/RAM Based SR/Track/Hang  Plus 1 Pipe Stage/TH_10 ==
  Din : Inport
  Track : Inport  Port=2
  Delay : xbsIndex_r4/Delay  rst=off  infoeditControl=Selection of Reset will increase slice count due to use of real FFs and instead of SRLs  en=off  latency=1  dbl_ovrd=off  reg_retiming=off  block_type=delay
      settings: block_version=12.2
  Mux : xbsIndex_r4/Mux  inputs=2  en=off  latency=0  precision=Full  arith_type=Unsigned  n_bits=16  bin_pt=14  quantization=Truncate  overflow=Wrap  dbl_ovrd=off  block_type=mux
      settings: block_version=12.2
  Dout : Outport
  wires:
  Track/1 -> Mux/1
  Delay/1 -> Mux/2
  Din/1 -> Mux/3, Delay/1
  Mux/1 -> Dout/1

== system Xcvr_SSB_AM_2p5/RX Filters D=8192/Decimating Filter DC Optimized in Accumulator Plus Pipelined Stage Control. Improved dynamic  range. /D=2 Bit Serial Filter Core with Piplined RAM Based SR/RAM Based SR/Track/Hang  Plus 1 Pipe Stage/TH_11 ==
  Din : Inport
  Track : Inport  Port=2
  Delay : xbsIndex_r4/Delay  rst=off  infoeditControl=Selection of Reset will increase slice count due to use of real FFs and instead of SRLs  en=off  latency=1  dbl_ovrd=off  reg_retiming=off  block_type=delay
      settings: block_version=12.2
  Mux : xbsIndex_r4/Mux  inputs=2  en=off  latency=0  precision=Full  arith_type=Unsigned  n_bits=16  bin_pt=14  quantization=Truncate  overflow=Wrap  dbl_ovrd=off  block_type=mux
      settings: block_version=12.2
  Dout : Outport
  wires:
  Mux/1 -> Dout/1
  Din/1 -> Delay/1, Mux/3
  Delay/1 -> Mux/2
  Track/1 -> Mux/1

== system Xcvr_SSB_AM_2p5/RX Filters D=8192/Decimating Filter DC Optimized in Accumulator Plus Pipelined Stage Control. Improved dynamic  range. /D=2 Bit Serial Filter Core with Piplined RAM Based SR/RAM Based SR/Track/Hang  Plus 1 Pipe Stage/TH_2 ==
  Din : Inport
  Track : Inport  Port=2
  Delay : xbsIndex_r4/Delay  rst=off  infoeditControl=Selection of Reset will increase slice count due to use of real FFs and instead of SRLs  en=off  latency=1  dbl_ovrd=off  reg_retiming=off  block_type=delay
      settings: block_version=12.2
  Mux : xbsIndex_r4/Mux  inputs=2  en=off  latency=0  precision=Full  arith_type=Unsigned  n_bits=16  bin_pt=14  quantization=Truncate  overflow=Wrap  dbl_ovrd=off  block_type=mux
      settings: block_version=12.2
  Dout : Outport
  wires:
  Track/1 -> Mux/1
  Delay/1 -> Mux/2
  Din/1 -> Mux/3, Delay/1
  Mux/1 -> Dout/1

== system Xcvr_SSB_AM_2p5/RX Filters D=8192/Decimating Filter DC Optimized in Accumulator Plus Pipelined Stage Control. Improved dynamic  range. /D=2 Bit Serial Filter Core with Piplined RAM Based SR/RAM Based SR/Track/Hang  Plus 1 Pipe Stage/TH_3 ==
  Din : Inport
  Track : Inport  Port=2
  Delay : xbsIndex_r4/Delay  rst=off  infoeditControl=Selection of Reset will increase slice count due to use of real FFs and instead of SRLs  en=off  latency=1  dbl_ovrd=off  reg_retiming=off  block_type=delay
      settings: block_version=12.2
  Mux : xbsIndex_r4/Mux  inputs=2  en=off  latency=0  precision=Full  arith_type=Unsigned  n_bits=16  bin_pt=14  quantization=Truncate  overflow=Wrap  dbl_ovrd=off  block_type=mux
      settings: block_version=12.2
  Dout : Outport
  wires:
  Mux/1 -> Dout/1
  Din/1 -> Delay/1, Mux/3
  Delay/1 -> Mux/2
  Track/1 -> Mux/1

== system Xcvr_SSB_AM_2p5/RX Filters D=8192/Decimating Filter DC Optimized in Accumulator Plus Pipelined Stage Control. Improved dynamic  range. /D=2 Bit Serial Filter Core with Piplined RAM Based SR/RAM Based SR/Track/Hang  Plus 1 Pipe Stage/TH_4 ==
  Din : Inport
  Track : Inport  Port=2
  Delay : xbsIndex_r4/Delay  rst=off  infoeditControl=Selection of Reset will increase slice count due to use of real FFs and instead of SRLs  en=off  latency=1  dbl_ovrd=off  reg_retiming=off  block_type=delay
      settings: block_version=12.2
  Mux : xbsIndex_r4/Mux  inputs=2  en=off  latency=0  precision=Full  arith_type=Unsigned  n_bits=16  bin_pt=14  quantization=Truncate  overflow=Wrap  dbl_ovrd=off  block_type=mux
      settings: block_version=12.2
  Dout : Outport
  wires:
  Track/1 -> Mux/1
  Delay/1 -> Mux/2
  Din/1 -> Mux/3, Delay/1
  Mux/1 -> Dout/1

== system Xcvr_SSB_AM_2p5/RX Filters D=8192/Decimating Filter DC Optimized in Accumulator Plus Pipelined Stage Control. Improved dynamic  range. /D=2 Bit Serial Filter Core with Piplined RAM Based SR/RAM Based SR/Track/Hang  Plus 1 Pipe Stage/TH_5 ==
  Din : Inport
  Track : Inport  Port=2
  Delay : xbsIndex_r4/Delay  rst=off  infoeditControl=Selection of Reset will increase slice count due to use of real FFs and instead of SRLs  en=off  latency=1  dbl_ovrd=off  reg_retiming=off  block_type=delay
      settings: block_version=12.2
  Mux : xbsIndex_r4/Mux  inputs=2  en=off  latency=0  precision=Full  arith_type=Unsigned  n_bits=16  bin_pt=14  quantization=Truncate  overflow=Wrap  dbl_ovrd=off  block_type=mux
      settings: block_version=12.2
  Dout : Outport
  wires:
  Mux/1 -> Dout/1
  Din/1 -> Delay/1, Mux/3
  Delay/1 -> Mux/2
  Track/1 -> Mux/1

== system Xcvr_SSB_AM_2p5/RX Filters D=8192/Decimating Filter DC Optimized in Accumulator Plus Pipelined Stage Control. Improved dynamic  range. /D=2 Bit Serial Filter Core with Piplined RAM Based SR/RAM Based SR/Track/Hang  Plus 1 Pipe Stage/TH_6 ==
  Din : Inport
  Track : Inport  Port=2
  Delay : xbsIndex_r4/Delay  rst=off  infoeditControl=Selection of Reset will increase slice count due to use of real FFs and instead of SRLs  en=off  latency=1  dbl_ovrd=off  reg_retiming=off  block_type=delay
      settings: block_version=12.2
  Mux : xbsIndex_r4/Mux  inputs=2  en=off  latency=0  precision=Full  arith_type=Unsigned  n_bits=16  bin_pt=14  quantization=Truncate  overflow=Wrap  dbl_ovrd=off  block_type=mux
      settings: block_version=12.2
  Dout : Outport
  wires:
  Track/1 -> Mux/1
  Delay/1 -> Mux/2
  Din/1 -> Mux/3, Delay/1
  Mux/1 -> Dout/1

== system Xcvr_SSB_AM_2p5/RX Filters D=8192/Decimating Filter DC Optimized in Accumulator Plus Pipelined Stage Control. Improved dynamic  range. /D=2 Bit Serial Filter Core with Piplined RAM Based SR/RAM Based SR/Track/Hang  Plus 1 Pipe Stage/TH_7 ==
  Din : Inport
  Track : Inport  Port=2
  Delay : xbsIndex_r4/Delay  rst=off  infoeditControl=Selection of Reset will increase slice count due to use of real FFs and instead of SRLs  en=off  latency=1  dbl_ovrd=off  reg_retiming=off  block_type=delay
      settings: block_version=12.2
  Mux : xbsIndex_r4/Mux  inputs=2  en=off  latency=0  precision=Full  arith_type=Unsigned  n_bits=16  bin_pt=14  quantization=Truncate  overflow=Wrap  dbl_ovrd=off  block_type=mux
      settings: block_version=12.2
  Dout : Outport
  wires:
  Mux/1 -> Dout/1
  Din/1 -> Delay/1, Mux/3
  Delay/1 -> Mux/2
  Track/1 -> Mux/1

== system Xcvr_SSB_AM_2p5/RX Filters D=8192/Decimating Filter DC Optimized in Accumulator Plus Pipelined Stage Control. Improved dynamic  range. /D=2 Bit Serial Filter Core with Piplined RAM Based SR/RAM Based SR/Track/Hang  Plus 1 Pipe Stage/TH_8 ==
  Din : Inport
  Track : Inport  Port=2
  Delay : xbsIndex_r4/Delay  rst=off  infoeditControl=Selection of Reset will increase slice count due to use of real FFs and instead of SRLs  en=off  latency=1  dbl_ovrd=off  reg_retiming=off  block_type=delay
      settings: block_version=12.2
  Mux : xbsIndex_r4/Mux  inputs=2  en=off  latency=0  precision=Full  arith_type=Unsigned  n_bits=16  bin_pt=14  quantization=Truncate  overflow=Wrap  dbl_ovrd=off  block_type=mux
      settings: block_version=12.2
  Dout : Outport
  wires:
  Track/1 -> Mux/1
  Delay/1 -> Mux/2
  Din/1 -> Mux/3, Delay/1
  Mux/1 -> Dout/1

== system Xcvr_SSB_AM_2p5/RX Filters D=8192/Decimating Filter DC Optimized in Accumulator Plus Pipelined Stage Control. Improved dynamic  range. /D=2 Bit Serial Filter Core with Piplined RAM Based SR/RAM Based SR/Track/Hang  Plus 1 Pipe Stage/TH_9 ==
  Din : Inport
  Track : Inport  Port=2
  Delay : xbsIndex_r4/Delay  rst=off  infoeditControl=Selection of Reset will increase slice count due to use of real FFs and instead of SRLs  en=off  latency=1  dbl_ovrd=off  reg_retiming=off  block_type=delay
      settings: block_version=12.2
  Mux : xbsIndex_r4/Mux  inputs=2  en=off  latency=0  precision=Full  arith_type=Unsigned  n_bits=16  bin_pt=14  quantization=Truncate  overflow=Wrap  dbl_ovrd=off  block_type=mux
      settings: block_version=12.2
  Dout : Outport
  wires:
  Mux/1 -> Dout/1
  Din/1 -> Delay/1, Mux/3
  Delay/1 -> Mux/2
  Track/1 -> Mux/1
